simulink model "IIRFilterDesign"  (R2023b)
settings: Solver=VariableStepAuto  StartTime=0.0  StopTime=10.0  RelTol=1e-3
settings Model: Creator=pratikmandi  LastModifiedBy=pratikmandi

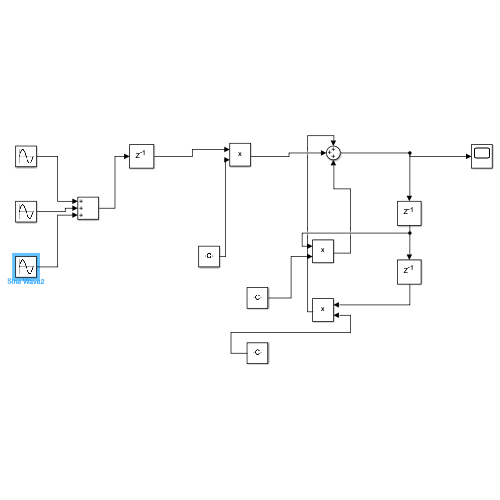
[thumbnail: Simulink's stored preview of the top-level diagram]
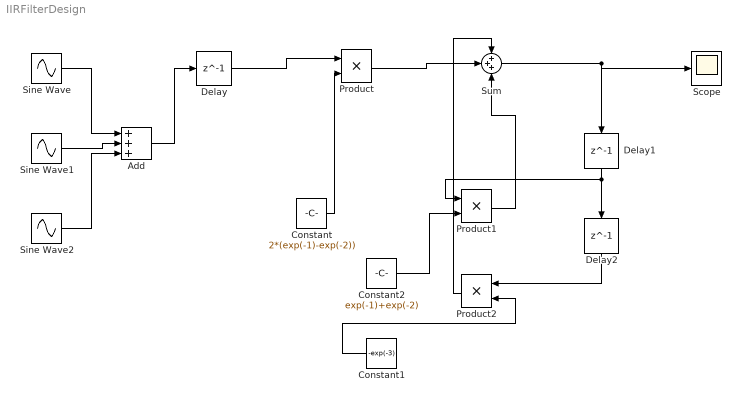
== system IIRFilterDesign ==
  Add : Sum  Inputs=+++
  Constant : Constant  Value=2*(exp(-1)-exp(-2))
  Constant1 : Constant  Value=-exp(-3)
  Constant2 : Constant  Value=exp(-1)+exp(-2)
  Delay : Delay  DelayLength=1
  Delay1 : Delay  DelayLength=1
  Delay2 : Delay  DelayLength=1
  Product : Product
  Product1 : Product
  Product2 : Product
  Scope : Scope
  Sine Wave : Sin  Frequency=10  SampleTime=0
  Sine Wave1 : Sin  Frequency=500  SampleTime=0
  Sine Wave2 : Sin  Frequency=2000  SampleTime=0
  Sum : Sum  Inputs=+++
  wires:
  Delay1/1 -> Delay2/1, Product1/1
  Sum/1 -> Scope/1, Delay1/1
  Product/1 -> Sum/2
  Sine Wave/1 -> Add/1
  Sine Wave1/1 -> Add/2
  Sine Wave2/1 -> Add/3
  Add/1 -> Delay/1
  Delay/1 -> Product/1
  Constant/1 -> Product/2
  Delay2/1 -> Product2/1
  Constant1/1 -> Product2/2
  Constant2/1 -> Product1/2
  Product1/1 -> Sum/3
  Product2/1 -> Sum/1
